simulink model "mfcMU"  (R2015a)
settings: Solver=ode15s  StartTime=0.0  StopTime=500  RelTol=1e-9  AbsTol=1e-12
InitFcn:
  | delta = 20;
  | kmu = 1000000;
  | 
  | beta = 0;
  | %beta = -10;
  | gamma = 0;
  | %gamma = 5;
  | 
  | dummy = 0;
  | 
  | %mfcInit = [5.726117682433310 0.030299840936202];
  | mfcInit1 = [2.176890899572858   0.049997860417195];
  | mfcInit2= [2.176961197280646   0.049996472695857];
values from neighbouring files (symbols this model uses):
  Rinit = 200    [mfcMUmodel.m]    (also in mfcMultiUnit.m)
settings Model: Creator=ironi  LastModifiedBy=ironi
settings HardwareCC: ProdBitPerLong=64  ProdBitPerPointer=64  ProdWordSize=64  ProdHWDeviceType=Generic->64-bit Embedded Processor (LP64)

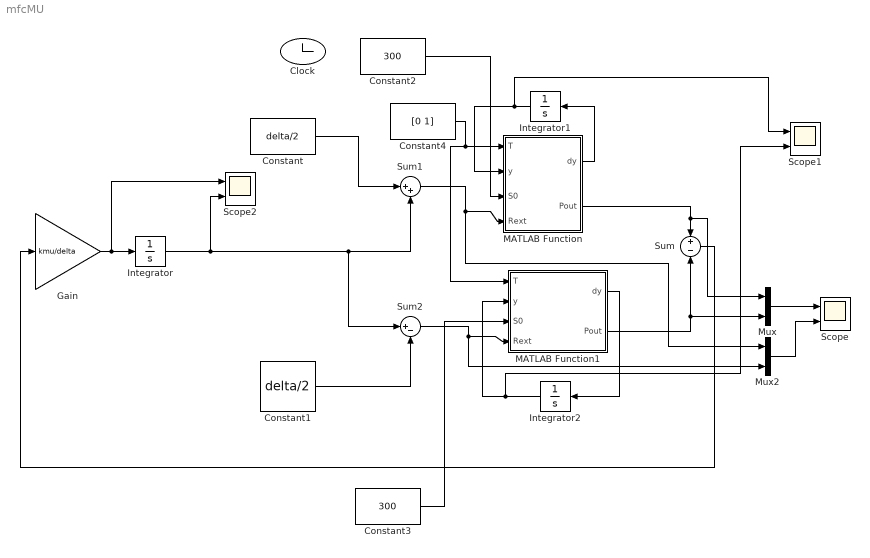
== system mfcMU ==
  Clock : Clock
  Constant : Constant  Value=delta/2
  Constant1 : Constant  Value=delta/2
  Constant2 : Constant  Value=300
  Constant3 : Constant  Value=300
  Constant4 : Constant  Value=[0 1]
  Gain : Gain  Gain=kmu/delta
  Integrator : Integrator  InitialCondition=Rinit
  Integrator1 : Integrator  InitialCondition=mfcInit2
  Integrator2 : Integrator  InitialCondition=mfcInit1
  MATLAB Function : MATLAB Function  TreatAsAtomicUnit=on
  MATLAB Function1 : MATLAB Function  TreatAsAtomicUnit=on
  Mux : Mux  Inputs=2
  Mux2 : Mux  Inputs=2
  Scope : Scope  NumInputPorts=2
      settings: YMin=0.00172~147  YMax=0.001734~168
  Scope1 : Scope  NumInputPorts=2
      settings: YMin=0.00172~147  YMax=0.001734~168
  Scope2 : Scope  NumInputPorts=2
      settings: YMin=0.00172~147  YMax=0.001734~168  SaveName=ScopeData2
  Sum : Sum  Inputs=+|-
  Sum1 : Sum  Inputs=|++
  Sum2 : Sum  Inputs=|+-
  wires:
  Sum/1 -> Gain/1
  Gain/1 -> Scope2/1, Integrator/1
  Sum1/1 -> MATLAB Function/4(Rext), Mux2/1
  Constant/1 -> Sum1/1
  Mux/1 -> Scope/1
  Constant1/1 -> Sum2/2
  Sum2/1 -> MATLAB Function1/4(Rext), Mux2/2
  MATLAB Function/1(dy) -> Integrator1/1
  Mux2/1 -> Scope/2
  MATLAB Function1/2(Pout) -> Mux/2, Sum/2
  MATLAB Function/2(Pout) -> Mux/1, Sum/1
  Integrator1/1 -> Scope1/1, MATLAB Function/2(y)
  MATLAB Function1/1(dy) -> Integrator2/1
  Constant4/1 -> MATLAB Function1/1(T), MATLAB Function/1(T)
  Constant2/1 -> MATLAB Function/3(S0)
  Constant3/1 -> MATLAB Function1/3(S0)
  Integrator/1 -> Scope2/2, Sum2/1, Sum1/2
  Integrator2/1 -> Scope1/2, MATLAB Function1/2(y)

== matlab function mfcMU/MATLAB Function1 ==
  data: T input; dy output; y input; dummy parameter; S0 input; Rext input; Pout output
function [dy, Pout]= mfcModelFast(T, y, dummy, S0, Rext)
F = 96485;%
R = 8.314472;%
T = 298.15;%
yield = 22.753;%
% Ych4 = .3;%
qmax_a = 8.484;%
qmax_m = 8.2;%
umax_a = 1.9753;%
umax_m = .1;%
Ks_a = 20;%
Ks_m = 80;%
m = 2;%
gamma = 663400;%
Mtotal = .05;%
Km = .2*Mtotal;%
% Kd_a = .02*umax_a;%
% Kd_m = .02*umax_m;%
Xmax = 512.5;%
Kx = .01*4;%
Rmin = 25;%
Rmax = 2000 + Rmin;%
Emin = .01;%
Emax = 0.25 + 0.4144+ Emin;%
Kr = .024;%

% i0ref=0.4*4;%

e = 0.0001*Mtotal;%

V = 0.2;%
Fin = 0.1527;%

D = Fin/V;

Xtot = 500;

Xeg = 250;

S   = y(1);
Mox = y(2);
xm = Xtot - Xeg;


%% Équations dynamiques
  
Mred = Mtotal - Mox;

Rint = Rmin + (Rmax - Rmin) * exp(-Kr*Xeg);                         % (22)
Eocv = Emin + (Emax - Emin) * exp(-1/(Kr*Xeg));                     % (23)

% alpha = 1/2*(1 + tanh(Kx*(Xeg + xm - Xmax)));                    % (9)

qa = qmax_a * S / (Ks_a + S) * Mox / (Km + Mox);                    % (15)
qm = qmax_m * S / (Ks_m + S);                                       % (16)

% ueg = umax_a * S / (Ks_a + S) * Mox / (Km + Mox);                    % (13)

% Imfc = (Eocv - n_conc) / (Rext + Rint) * Mred / (e + Mred);         % (21)
temp = Eocv - (R*T/m/F)*abs(log(complex(Mtotal/Mred)));
% Imfc = (Eocv - (R*T/m/F)*abs(log(complex(Mtotal/Mred))))/(Rext+Rint)*Mred/(e+Mred);
Imfc = temp/(Rext+Rint)*Mred/(e+Mred);

% Pout = ((Eocv - (R*T/m/F)*abs(log(complex(Mtotal/Mred))))*Mred/(e+Mred)-Rint*Imfc)*Imfc;
Pout = (temp*Mred/(e+Mred)-Rint*Imfc)*Imfc;

Sp = -qa*Xeg - qm*xm + D*(S0 - S);                                   % (6)
% Xap = ueg*xa - Kd_a*xa - alpha_a*D*xa;                               % (7)
% Xmp = um*xm - Kd_m*xm - alpha_m*D*xm;                               % (8)

Moxp = -yield*qa + gamma*Imfc / (m*F*V*Xeg) * 86400;                 % (12)

% if xa < 1 && Xap < 0
%   Xap = 0;
% end
% 
% if xm < 0.99 && Xmp < 0
%   Xmp = 0;
% end

% Pout = Rext*Imfc^2;

% dy = [Sp; Xap; Xmp; Moxp];
dy = [Sp; Moxp];

== matlab function mfcMU/MATLAB Function ==
  data: T input; dy output; y input; dummy parameter; S0 input; Rext input; Pout output
function [dy, Pout]= mfcModelFast(T, y, dummy, S0, Rext)
F = 96485;%
R = 8.314472;%
T = 298.15;%
yield = 22.753;%
% Ych4 = .3;%
qmax_a = 8.484;%
qmax_m = 8.2;%
umax_a = 1.9753;%
umax_m = .1;%
Ks_a = 20;%
Ks_m = 80;%
m = 2;%
gamma = 663400;%
Mtotal = .05;%
Km = .2*Mtotal;%
% Kd_a = .02*umax_a;%
% Kd_m = .02*umax_m;%
Xmax = 512.5;%
Kx = .01*4;%
Rmin = 25;%
Rmax = 2000 + Rmin;%
Emin = .01;%
Emax = 0.25 + 0.4144+ Emin;%
Kr = .024;%

% i0ref=0.4*4;%

e = 0.0001*Mtotal;%

V = 0.2;%
Fin = 0.1527;%

D = Fin/V;

Xtot = 500;

Xeg = 250;

S   = y(1);
Mox = y(2);
xm = Xtot - Xeg;


%% Équations dynamiques
  
Mred = Mtotal - Mox;

Rint = Rmin + (Rmax - Rmin) * exp(-Kr*Xeg);                         % (22)
Eocv = Emin + (Emax - Emin) * exp(-1/(Kr*Xeg));                     % (23)

% alpha = 1/2*(1 + tanh(Kx*(Xeg + xm - Xmax)));                    % (9)

qa = qmax_a * S / (Ks_a + S) * Mox / (Km + Mox);                    % (15)
qm = qmax_m * S / (Ks_m + S);                                       % (16)

% ueg = umax_a * S / (Ks_a + S) * Mox / (Km + Mox);                    % (13)

% Imfc = (Eocv - n_conc) / (Rext + Rint) * Mred / (e + Mred);         % (21)
temp = Eocv - (R*T/m/F)*abs(log(complex(Mtotal/Mred)));
% Imfc = (Eocv - (R*T/m/F)*abs(log(complex(Mtotal/Mred))))/(Rext+Rint)*Mred/(e+Mred);
Imfc = temp/(Rext+Rint)*Mred/(e+Mred);

% Pout = ((Eocv - (R*T/m/F)*abs(log(complex(Mtotal/Mred))))*Mred/(e+Mred)-Rint*Imfc)*Imfc;
Pout = (temp*Mred/(e+Mred)-Rint*Imfc)*Imfc;

Sp = -qa*Xeg - qm*xm + D*(S0 - S);                                   % (6)
% Xap = ueg*xa - Kd_a*xa - alpha_a*D*xa;                               % (7)
% Xmp = um*xm - Kd_m*xm - alpha_m*D*xm;                               % (8)

Moxp = -yield*qa + gamma*Imfc / (m*F*V*Xeg) * 86400;                 % (12)

% if xa < 1 && Xap < 0
%   Xap = 0;
% end
% 
% if xm < 0.99 && Xmp < 0
%   Xmp = 0;
% end

% Pout = Rext*Imfc^2;

% dy = [Sp; Xap; Xmp; Moxp];
dy = [Sp; Moxp];
